simulink model "BuckeyeCurrent_Simulation"  (R2018a)
settings: Solver=FixedStepAuto  StartTime=0.0  StopTime=Inf  MinStep=0.01  RelTol=1e-3
undefined symbols (not defined in the file): A1, AIR, ambTemp_K, BATT_ELEC, BATT_OCV, BATT_THERMAL, C1, C2, Cell, COOLANT, cp, Elevation_Profile, EM, flowrate, hA1, k12, M, M2, MOT, RAD, soc0, V_pack_init, Velocity_Profile
libraries: simulink x3
(part 1 of 2)
settings Model: Creator=salyer.103  LastModifiedBy=Zach
settings SolverCC: ZeroCrossAlgorithm=Adaptive
settings CodeAppCC: StateflowObjectComments=on

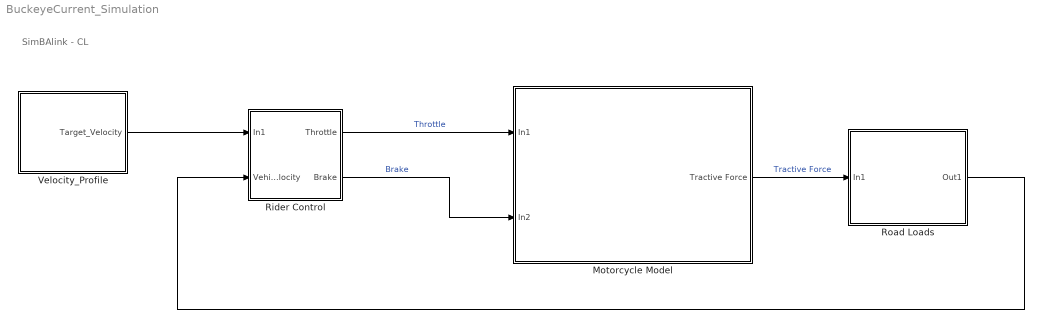
== system BuckeyeCurrent_Simulation ==
  note: SimBAlink - CL
  Motorcycle Model : Subsystem  mask{EM_MC_Selection=emrax268_pm150dz, SOC_max=0.95, SOC_min=0.10, Cell_Selection=Ideal, Wheel_Radius=0.3, Final_Drive_Eff=0.92, Max_Brake_Torque=4000, Total_Mass=330, b=0.728, h=0.72, g=9.81, p=1.4, mu_r=1, Front_Sprocket=21, Rear_Sprocket_FirstGear=40, Rear_Sprocket_SecondGear=40, Regen_Percent=0, Whl_Inertia=0, Transmission_Inertia=0}
      mask prompts: EM_MC_Selection "Motor & Controller Selection"; SOC_max "Maximum SOC"; SOC_min "Minimum SOC"; Cell_Selection "Cell Selection"; Wheel_Radius "Wheel Radius (m)"; Final_Drive_Eff "Efficiency of Drivetrain"; Max_Brake_Torque "Maximum Braking Torque (Nm)"; Total_Mass "Vehicle Total Mass (kg)"; b "Distance from Rear Wheel to CG (m)"; h "Height of CG from ground (m)"; g "Gravity (m/s2)"; p "Wheelbase (m)"; mu_r "Rear Wheel Coefficient of Friction"; Front_Sprocket "Front Sprocket Teeth"; Rear_Sprocket_FirstGear "Rear Sprocket 1st"; Rear_Sprocket_SecondGear "Rear Sprocket 2nd"; Regen_Percent "Percentage of Max Regen (%)"; Whl_Inertia "Wheel Inertia (kg-m2)"; Transmission_Inertia "Transmission Inertia (kg-m2)"
      mask init:
      | Initialize_Powertrain
      | Initialize_BatteryPack
      mask TypeOptions EM_MC_Selection: emrax268_pm150dz | RemyHVH25090s | emrax228_Twin | Ideal_TomegaCurve
      mask TypeOptions Cell_Selection: Ideal | Efest_IMR18650 | LG_INR18650HG2 | LG_INR18650MJ1 | SanPan_NCR18650GA
      mask Display:
      | directory = pwd;
      | image([pwd '\Mask Pictures\bike.jpg']);
  Rider Control : Subsystem  mask{kp=5, ki=0, kd=0}
      mask Display:
      | directory = pwd;
      | image([pwd '\Mask Pictures\helmet.jpg']);
  Road Loads : Subsystem  mask{rowA=1, Wind_Speed=0, Cda=0.38, ElevationProfile=IOM_ElevationProfile}
      mask prompts: rowA "Air Density"; Wind_Speed "Wind Speed (m/s)"; Cda "Cd * Frontal Area"; ElevationProfile "Course Elevation Profile"
      mask init:
      | Initialize_Elevation
      mask TypeOptions ElevationProfile: IOM_ElevationProfile | QuarterMile_ElevationProfile
  Velocity_Profile : Subsystem  mask{Circuit_Selection=IOM}
      mask prompts: Circuit_Selection "Circuit"
      mask init:
      | Initialize_Circuit
      mask TypeOptions Circuit_Selection: IOM | QuarterMile
      mask Display:
      | directory = pwd;
      | image([pwd '\Mask Pictures\VelocityProfile.png']);
  wires:
  Velocity_Profile/1(Target_Velocity) -> Rider Control/1(In1)
  Rider Control/1(Throttle) -> Motorcycle Model/1(In1)  "Throttle"
  Rider Control/2(Brake) -> Motorcycle Model/2(In2)  "Brake"
  Motorcycle Model/1(Tractive Force) -> Road Loads/1(In1)  "Tractive Force"
  Road Loads/1(Out1) -> Rider Control/2(Vehicle_Velocity)

== system BuckeyeCurrent_Simulation/Motorcycle Model ==
  note: When Rear Braking Strategy is added, will need to move pack energy req block
      | B/c negative torque applied gives regen to pack
      |
      | To determine actual applied torque prior to the wheel block we will  need to modulate torque based on
      | wheel slip from the rider model
  In1 : Inport
  In2 : Inport  Port=2
  Battery Pack : Subsystem
      mask Display:
      | directory = pwd;
      | image([directory '\Mask Pictures\pack.JPG']);
  Braking/Throttle Strategy : Subsystem
  Front Brakes : Subsystem
      mask Display:
      | directory = pwd;
      | image([directory '\Mask Pictures\motoBrake.JPG']);
  Front Wheel (Force Limits) : Subsystem
      mask Display:
      | directory = pwd;
      | image([directory '\Mask Pictures\frTire_pirelli.JPG']);
  Powertrain : Subsystem
      mask Display:
      | directory = pwd;
      | image([directory '\Mask Pictures\bike_powertrain.JPG']);
  Rear Brakes : Subsystem
      mask Display:
      | directory = pwd;
      | image([directory '\Mask Pictures\motoBrake.JPG']);
  Rear Wheel (Force Limits) : Subsystem
      mask Display:
      | directory = pwd;
      | image([directory '\Mask Pictures\rrTire_pirelli.JPG']);
  Sum : Sum  Inputs=+|+
  Sum1 : Sum  Inputs=++|
  To Workspace : ToWorkspace  VariableName=RearWhlForce  SampleTime=-1
  To Workspace1 : ToWorkspace  VariableName=FrontWhlForce  SaveFormat=Timeseries  SampleTime=-1
  Transmission : Subsystem
      mask Display:
      | directory = pwd;
      | image([directory '\Mask Pictures\gear.PNG']);
  Vehicle Parameters : Subsystem
  Tractive Force : Outport
  wires:
  Sum/1 -> Tractive Force/1  "Tractive Force"
  Powertrain/1(Motor Torque) -> Transmission/1(Motor Torque)
  Front Brakes/1(Front Wheel Torque) -> Front Wheel (Force Limits)/1(In1)
  Front Wheel (Force Limits)/1(Out2) -> Sum/1, To Workspace1/1
  Rear Wheel (Force Limits)/1(Out1) -> Sum/2, To Workspace/1
  In1/1 -> Braking/Throttle Strategy/1(In1)  "Throttle"
  Braking/Throttle Strategy/3(Out2) -> Powertrain/1(Throttle)
  In2/1 -> Braking/Throttle Strategy/2(In2)  "Brake"
  Braking/Throttle Strategy/1(Out3) -> Front Brakes/1(Throttle)
  Transmission/1(Out1) -> Sum1/2  "Wheel Torque"
  Rear Brakes/1(Front Wheel Torque) -> Sum1/1  "Rear Brake Torque"
  Sum1/1 -> Rear Wheel (Force Limits)/1(In1)  "Total Torque"
  Braking/Throttle Strategy/2(Out1) -> Rear Brakes/1(Throttle)
  Powertrain/2(Out1) -> Battery Pack/1(In1)  "Power Request"
  Battery Pack/1(Power Limit) -> Powertrain/2(df\)  "Power Limit"
  Battery Pack/2(Power Limit1) -> Powertrain/3(df\1)  "Terminal Voltage"

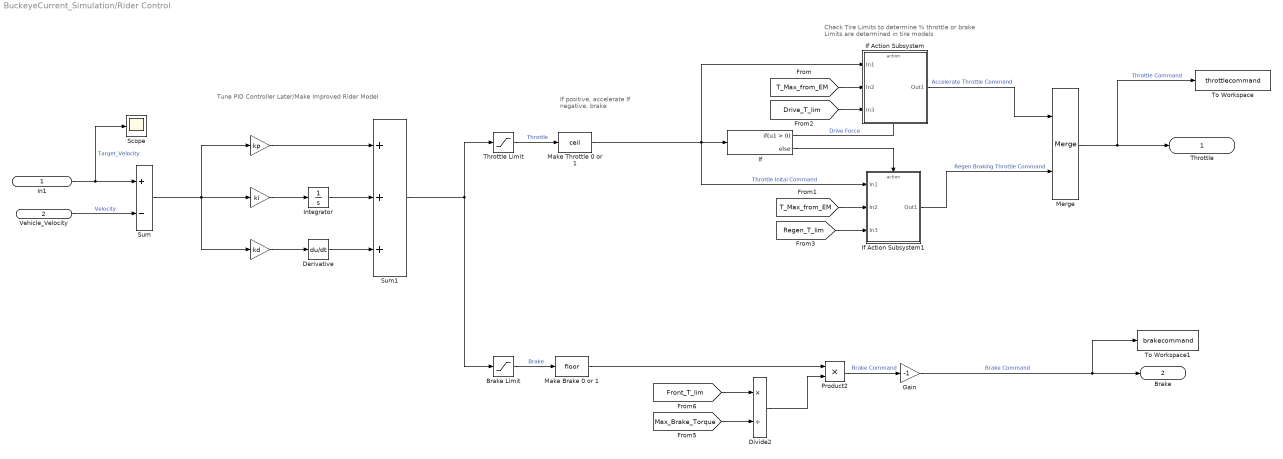
== system BuckeyeCurrent_Simulation/Rider Control ==
  note: Check Tire Limits to determine % throttle or brake
      | Limits are determined in tire models
  note: If positive, accelerate
      | If negative, brake
  note: Tune PID Controller Later/Make Improved Rider Model
  In1 : Inport
  Vehicle_Velocity : Inport  Port=2
  " " : Gain  Gain=ki
  "  " : Gain  Gain=kp
  "   " : Gain  Gain=kd
  Brake Limit : Saturate  UpperLimit=0  LowerLimit=-1  ZeroCross=off
  Derivative : Derivative
  Divide2 : Product  Inputs=*/
  Gain : Gain  Gain=-1
  If : If
  If Action Subsystem : Subsystem  TreatAsAtomicUnit=on
  If Action Subsystem1 : Subsystem  TreatAsAtomicUnit=on
  Integrator : Integrator
  Make Brake 0 or 1 : Rounding
  Make Throttle 0 or 1 : Rounding  Operator=ceil
  Merge : Merge
  Product2 : Product
  Scope : Scope
  Sum : Sum  Inputs=+-
  Sum1 : Sum  Inputs=+++
  Throttle Limit : Saturate  UpperLimit=1  LowerLimit=0  ZeroCross=off
  To Workspace : ToWorkspace  VariableName=throttlecommand  SampleTime=-1
  To Workspace1 : ToWorkspace  VariableName=brakecommand  SampleTime=-1
  Throttle : Outport
  Brake : Outport  Port=2
  wires:
  Vehicle_Velocity/1 -> Sum/2  "Velocity"
  In1/1 -> Scope/1, Sum/1  "Target_Velocity"
  "  "/1 -> Sum1/1
  Sum/1 -> "  "/1, " "/1, "   "/1
  Throttle Limit/1 -> Make Throttle 0 or 1/1  "Throttle"
  " "/1 -> Integrator/1
  Integrator/1 -> Sum1/2
  "   "/1 -> Derivative/1
  Derivative/1 -> Sum1/3
  Sum1/1 -> Brake Limit/1, Throttle Limit/1
  Brake Limit/1 -> Make Brake 0 or 1/1  "Brake"
  Make Throttle 0 or 1/1 -> If Action Subsystem/1(In1), If Action Subsystem1/1(In1), If/1  "Throttle Inital Command"
  Merge/1 -> To Workspace/1, Throttle/1  "Throttle Command"
  [Max_Brake_Torque] -> Divide2/2
  [Front_T_lim] -> Divide2/1
  Divide2/1 -> Product2/2
  Make Brake 0 or 1/1 -> Product2/1
  Gain/1 -> To Workspace1/1, Brake/1  "Brake Command"
  If Action Subsystem/1(Out1) -> Merge/1  "Accelerate Throttle Command"
  If Action Subsystem1/1(Out1) -> Merge/2  "Regen Braking Throttle Command"
  [T_Max_from_EM] -> If Action Subsystem/2(In2)
  [T_Max_from_EM] -> If Action Subsystem1/2(In2)
  [Drive_T_lim] -> If Action Subsystem/3(In3)
  [Regen_T_lim] -> If Action Subsystem1/3(In3)
  If/1 -> If Action Subsystem/Action  "Drive Force"
  If/2 -> If Action Subsystem1/Action
  Product2/1 -> Gain/1  "Brake Command"

== system BuckeyeCurrent_Simulation/Road Loads ==
  In1 : Inport
  Enviornment : Subsystem
  To Workspace : ToWorkspace  VariableName=Vehicle_Velocity  SampleTime=-1
      settings: Save2DSignal=2-D array (concatenate along first dimension)
  To Workspace1 : ToWorkspace  VariableName=resistanceforce  SampleTime=-1
      settings: Save2DSignal=2-D array (concatenate along first dimension)
  Vehicle Loads : Subsystem
  Vehicle_speed_Calculation : Subsystem
  Out1 : Outport
  tag scope: Vehicle_Velocity_ms=global
  wires:
  In1/1 -> Vehicle_speed_Calculation/1(In1)  "Tractive Force"
  Vehicle_speed_Calculation/1(F (N)1) -> To Workspace/1, Out1/1, [Vehicle_Velocity_ms]  "Velocity"
  Vehicle Loads/1(F (N)) -> To Workspace1/1, Vehicle_speed_Calculation/2(In3)

== system BuckeyeCurrent_Simulation/Velocity_Profile ==
  Constant : Constant  Value=Velocity_Profile.distance(end)
  Relational Operator1 : RelationalOperator  RndMeth=Nearest  InputSameDT=on
  Stop Simulation : Stop
  To Workspace : ToWorkspace  VariableName=Target_Velocity  SampleTime=-1
  Vehicle_Target_Speed : Lookup  InputValues=Velocity_Profile.distance  Table=Velocity_Profile.velocity  LookUpMeth=Interpolation-Use End Values  SaturateOnIntegerOverflow=on
  Target_Velocity : Outport
  wires:
  Vehicle_Target_Speed/1 -> To Workspace/1, Target_Velocity/1  "Target_Velocity"
  Constant/1 -> Relational Operator1/2
  Relational Operator1/1 -> Stop Simulation/1
  [Distance_Total_m] -> Relational Operator1/1, Vehicle_Target_Speed/1

== system BuckeyeCurrent_Simulation/Motorcycle Model/Battery Pack ==
  In1 : Inport
  0th Order Cell Model : Subsystem
  Constant : Constant  Value=Cell.Np
  Constant2 : Constant  Value=Cell.Ns
  Constant3 : Constant  Value=Cell.Nt
  "Current Lim, 1st Order ECM, Thermal, Regen" : Subsystem  Commented=on
  Integrator : Integrator
  Multiply : Product  Inputs=*/
  Multiply1 : Product  Inputs=*/
  Multiply{2..4,6} (4 alike) : Product
  To Workspace1 : ToWorkspace  VariableName=P_pack  SampleTime=-1
      settings: Save2DSignal=2-D array (concatenate along first dimension)
  To Workspace2 : ToWorkspace  VariableName=E_pack  SampleTime=-1
      settings: Save2DSignal=2-D array (concatenate along first dimension)
  To Workspace3 : ToWorkspace  VariableName=I_pack  SampleTime=-1
      settings: Save2DSignal=2-D array (concatenate along first dimension)
  To Workspace4 : ToWorkspace  VariableName=SOC  SampleTime=-1
      settings: Save2DSignal=2-D array (concatenate along first dimension)
  To Workspace5 : ToWorkspace  VariableName=V_pack  SampleTime=-1
      settings: Save2DSignal=2-D array (concatenate along first dimension)
  To Workspace6 : ToWorkspace  VariableName=Q_pack  SampleTime=-1
      settings: Save2DSignal=2-D array (concatenate along first dimension)
  W to kW : Gain  Gain=1/1000
  kW-s to kW-h : Gain  Gain=1/3600
  Power Limit : Outport
  Power Limit1 : Outport  Port=2
  wires:
  kW-s to kW-h/1 -> To Workspace2/1
  Integrator/1 -> kW-s to kW-h/1  "Energy"
  W to kW/1 -> Integrator/1, To Workspace1/1
  Multiply1/1 -> 0th Order Cell Model/1(Current [A])
  Multiply/1 -> Multiply1/1, Multiply6/1, To Workspace3/1
  Constant/1 -> Multiply1/2
  In1/1 -> Multiply/1  "Inverter_Power_Request"
  0th Order Cell Model/1(SOC [-]) -> To Workspace4/1
  0th Order Cell Model/3(Heat Generation [W]) -> Multiply2/1
  Constant3/1 -> Multiply2/2, Multiply4/2
  0th Order Cell Model/4(" Cell Voltage [V]") -> Multiply3/1
  Constant2/1 -> Multiply3/2
  Multiply3/1 -> Power Limit1/1, To Workspace5/1, Multiply6/2, Multiply/2  "Terminal Voltage"
  Multiply2/1 -> To Workspace6/1
  Multiply4/1 -> Power Limit/1  "Power Limit"
  0th Order Cell Model/2(Power Limit [W]) -> Multiply4/1
  Multiply6/1 -> W to kW/1

== system BuckeyeCurrent_Simulation/Motorcycle Model/Braking//Throttle Strategy ==
  note: Notes:
      | -No Rear Brake currently being used, no point in using it until we have a better rider model
      | -If throttle = 0, then switch to -1 to request negative torque
      | -Need to add a limit to rear brake force based on friction
  In1 : Inport
  In2 : Inport  Port=2
  Constant : Constant  Value=0
  Constant1 : Constant  Value=-1
  Gain : Gain
  Switch : Switch  Criteria=u2 > Threshold
  Out3 : Outport
  Out1 : Outport  Port=2
  Out2 : Outport  Port=3
  wires:
  Constant/1 -> Out1/1  "Rear Brake Request"
  In1/1 -> Switch/1, Switch/2  "Throttle Request"
  In2/1 -> Gain/1  "Brake Request"
  Gain/1 -> Out3/1  "Front Brake Request"
  Constant1/1 -> Switch/3
  Switch/1 -> Out2/1  "Torque Request"

== system BuckeyeCurrent_Simulation/Motorcycle Model/Front Brakes ==
  Throttle : Inport
  Multiply : Product  Inputs=**
  Front Wheel Torque : Outport
  wires:
  Throttle/1 -> Multiply/1  "Brake"
  [Max_Brake_Torque] -> Multiply/2
  Multiply/1 -> Front Wheel Torque/1  "Front Wheel Torque"

== system BuckeyeCurrent_Simulation/Motorcycle Model/Front Wheel (Force Limits) ==
  In1 : Inport
  Divide : Product  Inputs=*/
  Divide1 : Product  Inputs=**
  Dynamic Front Wheel Load * mu : Fcn  Expr=-mu_r*Total_Mass*g*b/p + u(1)*h/p
  Memory : Memory
  Memory1 : Memory
  Min : MinMax  Inputs=2
  Stoppie Limit Brake Force : Constant  Value=-Total_Mass*g*(p-b)/h
  Sum : Sum  Inputs=|++
  Sum1 : Sum
  Out2 : Outport
  tag scope: Front_Brake_Force=global, Front_T_lim=global
  wires:
  In1/1 -> Divide/1  "Front Wheel Torque"
  Divide/1 -> Out2/1, [Front_Brake_Force]  "Tractive Force"
  [Fr_Wheel_Radius] -> Divide/2
  Sum1/1 -> Dynamic Front Wheel Load * mu/1
  Dynamic Front Wheel Load * mu/1 -> Min/1
  Stoppie Limit Brake Force/1 -> Min/2
  [Front_Brake_Force] -> Memory/1
  Memory/1 -> Sum1/1
  Memory1/1 -> Sum1/2
  Min/1 -> Divide1/1
  Divide1/1 -> [Front_T_lim]
  [Fr_Wheel_Radius] -> Divide1/2
  Sum/1 -> Memory1/1
  [Regen_Brake_Force] -> Sum/1
  [Rear_Brake_Force] -> Sum/2

== system BuckeyeCurrent_Simulation/Motorcycle Model/Powertrain ==
  note: Note: Once thermal models are calibrated, the torque request will pass through those models to see if thermal is limiting power
      | -For now, assuming ideal motor and inverter
  Throttle : Inport
  df\ : Inport  Port=2
  df\1 : Inport  Port=3
  Divide : Product  Inputs=*/
  Gain : Gain  Gain=2*pi/60
  Integrator : Integrator
  Powertrain Mechanical : Subsystem
  Powertrain Thermal Model : Subsystem  Commented=on
  Product : Product
  Sum : Sum  Inputs=|-+
  To Workspace : ToWorkspace  VariableName=Heat_Energy_J  SampleTime=-1
  Motor Torque : Outport
  Out1 : Outport  Port=2
  wires:
  Throttle/1 -> Powertrain Mechanical/1(In1)  "Throttle"
  Powertrain Thermal Model/1(Out1) -> ?  "Motor Torque (With Possible Thermal Limtis)"
  Powertrain Thermal Model/2(Out2) -> ?  "Inverter_P_Request"
  Powertrain Mechanical/1(Out1) -> Product/1, Motor Torque/1  "Motor Torque"
  Powertrain Mechanical/2(EM RPM) -> Gain/1
  Gain/1 -> Product/2  "rad/s"
  Product/1 -> Sum/1, Divide/1  "Motor_Power_req"
  [EM_eff] -> Divide/2
  Divide/1 -> Sum/2, Out1/1  "Total_Power"
  Sum/1 -> Integrator/1  "heat_power_W"
  Integrator/1 -> To Workspace/1
  df\/1 -> Powertrain Mechanical/2(Power Limit)  "Power Limit"
  df\1/1 -> Powertrain Mechanical/3(Terminal Voltage)  "Terminal Voltage"

== system BuckeyeCurrent_Simulation/Motorcycle Model/Rear Brakes ==
  Throttle : Inport
  Multiply : Product  Inputs=**
  Front Wheel Torque : Outport
  tag scope: Rear_Brake_Force=global
  wires:
  Throttle/1 -> Multiply/1  "Brake"
  [Max_Brake_Torque] -> Multiply/2
  Multiply/1 -> [Rear_Brake_Force], Front Wheel Torque/1  "Rear Wheel Torque"

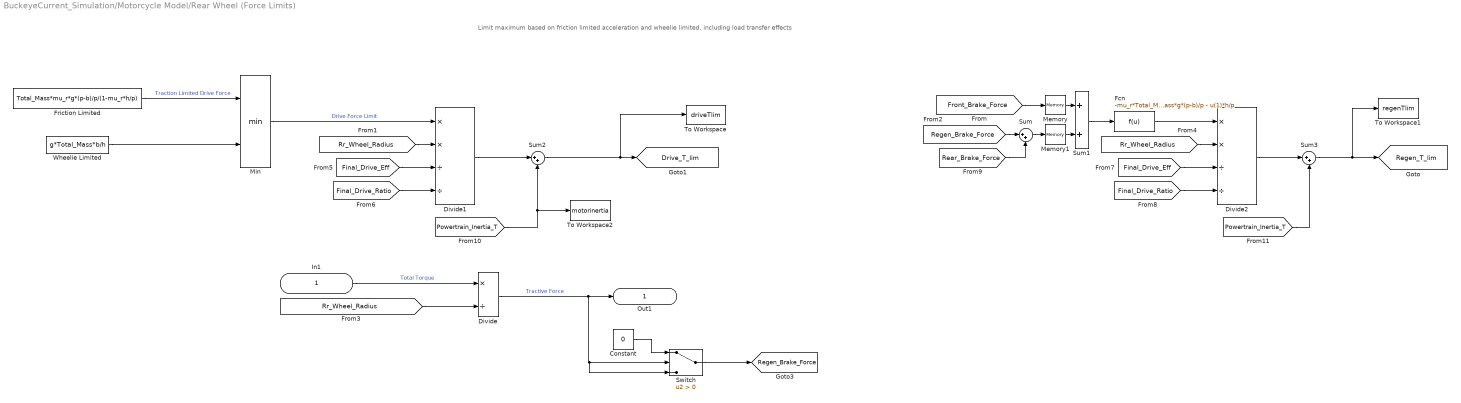
== system BuckeyeCurrent_Simulation/Motorcycle Model/Rear Wheel (Force Limits) ==
  note: Limit maximum based on friction limited acceleration and wheelie limited, including load transfer effects
  In1 : Inport
  Constant : Constant  Value=0
  Divide : Product  Inputs=*/
  Divide1 : Product  Inputs=**//
  Divide2 : Product  Inputs=**//
  Fcn : Fcn  Expr=-mu_r*Total_Mass*g*(p-b)/p - u(1)*h/p
  Friction Limited : Constant  Value=Total_Mass*mu_r*g*(p-b)/p/(1-mu_r*h/p)
  Memory : Memory
  Memory1 : Memory
  Min : MinMax  Inputs=2
  Sum : Sum  Inputs=|++
  Sum1 : Sum
  Sum2 : Sum  Inputs=|++
  Sum3 : Sum  Inputs=|++
  Switch : Switch  Criteria=u2 > Threshold
  To Workspace : ToWorkspace  VariableName=driveTlim  SampleTime=-1
  To Workspace1 : ToWorkspace  VariableName=regenTlim  SampleTime=-1
  To Workspace2 : ToWorkspace  VariableName=motorinertia  SampleTime=-1
  Wheelie Limited : Constant  Value=g*Total_Mass*b/h
  Out1 : Outport
  tag scope: Drive_T_lim=global, Regen_Brake_Force=global, Regen_T_lim=global
  wires:
  [Rr_Wheel_Radius] -> Divide/2
  Wheelie Limited/1 -> Min/2
  In1/1 -> Divide/1  "Total Torque"
  Divide/1 -> Switch/3, Switch/2, Out1/1  "Tractive Force"
  Sum1/1 -> Fcn/1
  Friction Limited/1 -> Min/1  "Traction Limited Drive Force"
  Min/1 -> Divide1/1  "Drive Force Limit"
  [Front_Brake_Force] -> Memory/1
  Memory/1 -> Sum1/1
  Memory1/1 -> Sum1/2
  Switch/1 -> [Regen_Brake_Force]
  Sum2/1 -> To Workspace/1, [Drive_T_lim]
  Fcn/1 -> Divide2/1
  Constant/1 -> Switch/1
  [Rr_Wheel_Radius] -> Divide1/2
  [Final_Drive_Eff] -> Divide1/3
  [Final_Drive_Ratio] -> Divide1/4
  [Final_Drive_Ratio] -> Divide2/4
  [Rr_Wheel_Radius] -> Divide2/2
  [Final_Drive_Eff] -> Divide2/3
  Sum/1 -> Memory1/1
  [Regen_Brake_Force] -> Sum/1
  [Rear_Brake_Force] -> Sum/2
  Divide1/1 -> Sum2/1
  [Powertrain_Inertia_T] -> To Workspace2/1, Sum2/2
  Divide2/1 -> Sum3/1
  Sum3/1 -> To Workspace1/1, [Regen_T_lim]
  [Powertrain_Inertia_T] -> Sum3/2

== system BuckeyeCurrent_Simulation/Motorcycle Model/Transmission ==
  note: Actual Motor RPM Depends on what gear we're in
  Motor Torque : Inport
  "CONVERT TO whl RPM " : Gain  Gain=60
  Calc wheel circumference : Gain  Gain=2*3.14
  Derivative : Derivative
  Gain : Gain  Gain=2*pi/60
  "Gearbox " : Subsystem
  To Workspace : ToWorkspace  VariableName=FinalDriveRatio  SampleTime=-1
      settings: Save2DSignal=2-D array (concatenate along first dimension)
  To Workspace1 : ToWorkspace  VariableName=RearWheelTorque  SampleTime=-1
      settings: Save2DSignal=2-D array (concatenate along first dimension)
  "convert to whl rev per sec " : Product  Inputs=*/
  "product rpm " : Product  Inputs=**
  product rpm 1 : Product  Inputs=**
  product rpm 2 : Product  Inputs=**
  Out1 : Outport
  tag scope: EM_RPM=global, EM_RPM_1st=global, EM_RPM_2nd=global, EM_acc=global
  wires:
  "Gearbox "/2(Out1) -> To Workspace1/1, Out1/1  "Rear Wheel Torque"
  Calc wheel circumference/1 -> "convert to whl rev per sec "/2
  [Vehicle_Velocity_ms] -> "convert to whl rev per sec "/1
  [Rr_Wheel_Radius] -> Calc wheel circumference/1
  "convert to whl rev per sec "/1 -> "CONVERT TO whl RPM "/1
  "product rpm "/1 -> Gain/1, [EM_RPM]
  Motor Torque/1 -> "Gearbox "/1(In1)  "Motor Torque"
  "CONVERT TO whl RPM "/1 -> product rpm 2/2, product rpm 1/2, "product rpm "/1
  [Final_Drive_Ratio_1st] -> product rpm 1/1
  [Final_Drive_Ratio_2nd] -> product rpm 2/1
  product rpm 1/1 -> [EM_RPM_1st]
  product rpm 2/1 -> [EM_RPM_2nd]
  "Gearbox "/1(Out2) -> To Workspace/1, "product rpm "/2
  Gain/1 -> Derivative/1  "EMl speed (rad/s)"
  Derivative/1 -> [EM_acc]

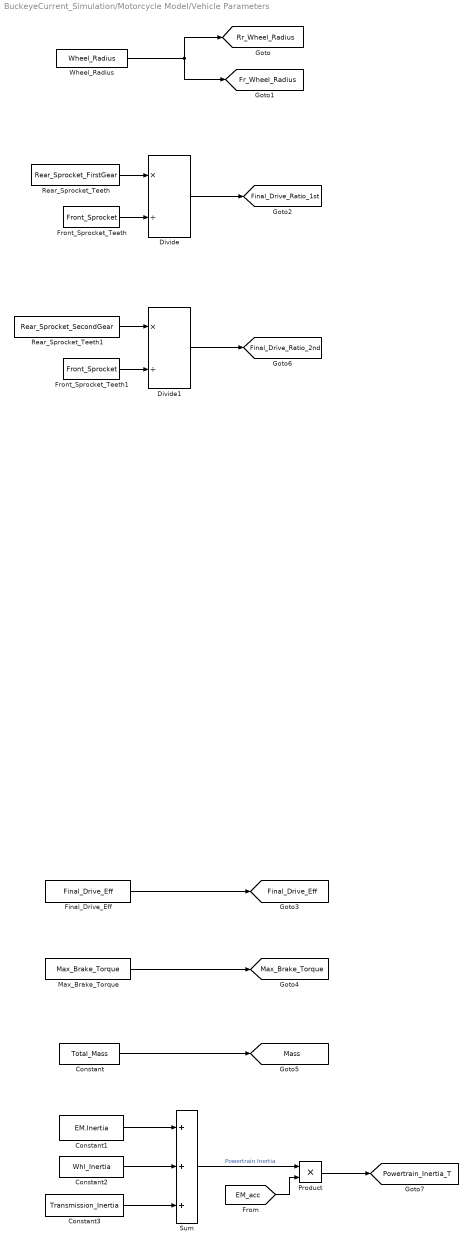
== system BuckeyeCurrent_Simulation/Motorcycle Model/Vehicle Parameters ==
  Constant : Constant  Value=Total_Mass
  Constant1 : Constant  Value=EM.Inertia
  Constant2 : Constant  Value=Whl_Inertia
  Constant3 : Constant  Value=Transmission_Inertia
  Divide : Product  Inputs=*/
  Divide1 : Product  Inputs=*/
  Final_Drive_Eff : Constant  Value=Final_Drive_Eff
  Front_Sprocket_Teeth : Constant  Value=Front_Sprocket
  Front_Sprocket_Teeth1 : Constant  Value=Front_Sprocket
  Max_Brake_Torque : Constant  Value=Max_Brake_Torque
  Product : Product
  Rear_Sprocket_Teeth : Constant  Value=Rear_Sprocket_FirstGear
  Rear_Sprocket_Teeth1 : Constant  Value=Rear_Sprocket_SecondGear
  Sum : Sum  Inputs=+++
  Wheel_Radius : Constant  Value=Wheel_Radius
  tag scope: Final_Drive_Eff=global, Final_Drive_Ratio_1st=global, Final_Drive_Ratio_2nd=global, Fr_Wheel_Radius=global, Mass=global, Max_Brake_Torque=global, Powertrain_Inertia_T=global, Rr_Wheel_Radius=global
  wires:
  Wheel_Radius/1 -> [Rr_Wheel_Radius], [Fr_Wheel_Radius]
  Front_Sprocket_Teeth/1 -> Divide/2
  Rear_Sprocket_Teeth/1 -> Divide/1
  Final_Drive_Eff/1 -> [Final_Drive_Eff]
  Max_Brake_Torque/1 -> [Max_Brake_Torque]
  Constant/1 -> [Mass]
  Divide/1 -> [Final_Drive_Ratio_1st]
  Divide1/1 -> [Final_Drive_Ratio_2nd]
  Rear_Sprocket_Teeth1/1 -> Divide1/1
  Front_Sprocket_Teeth1/1 -> Divide1/2
  Constant1/1 -> Sum/1
  Constant2/1 -> Sum/2
  Constant3/1 -> Sum/3
  Sum/1 -> Product/1  "Powertrain Inertia"
  [EM_acc] -> Product/2
  Product/1 -> [Powertrain_Inertia_T]

== system BuckeyeCurrent_Simulation/Rider Control/If Action Subsystem ==
  In1 : Inport
  In2 : Inport  Port=2
  In3 : Inport  Port=3
  Action Port : ActionPort  ActionType=then
  Divide : Product  Inputs=*/
  Product : Product
  Throttle Limit1 : Saturate  UpperLimit=1  LowerLimit=0  ZeroCross=off
  Out1 : Outport
  wires:
  Throttle Limit1/1 -> Out1/1
  Divide/1 -> Product/1
  In3/1 -> Divide/1
  In2/1 -> Divide/2  "T_Max_EM"
  In1/1 -> Product/2  "Drive Force"
  Product/1 -> Throttle Limit1/1

== system BuckeyeCurrent_Simulation/Rider Control/If Action Subsystem1 ==
  In1 : Inport
  In2 : Inport  Port=2
  In3 : Inport  Port=3
  Action Port : ActionPort  ActionType=else
  Constant : Constant  Value=-1
  Divide1 : Product  Inputs=*/
  Product1 : Product
  Sum2 : Sum  Inputs=|++
  Throttle Limit2 : Saturate  UpperLimit=0  LowerLimit=-1  ZeroCross=off
  Out1 : Outport
  wires:
  Throttle Limit2/1 -> Out1/1
  In1/1 -> Sum2/1
  Sum2/1 -> Product1/1  "Set throttle to -1"
  Constant/1 -> Sum2/2
  In3/1 -> Divide1/1
  Product1/1 -> Throttle Limit2/1
  In2/1 -> Divide1/2  "T_Max_EM"
  Divide1/1 -> Product1/2

== system BuckeyeCurrent_Simulation/Road Loads/Enviornment ==
  Constant : Constant  Value=Cda
  Constant1 : Constant  Value=Wind_Speed
  Constant4 : Constant  Value=rowA
  tag scope: Cda=global, Row_Air=global, Wind_Speed=global
  wires:
  Constant1/1 -> [Wind_Speed]  "wind speed"
  Constant4/1 -> [Row_Air]  "air density"
  Constant/1 -> [Cda]

== system BuckeyeCurrent_Simulation/Road Loads/Vehicle Loads ==
  Aerodynamic  Drag : Subsystem
  Grade Force : Subsystem
  Roll Force : Subsystem
  Sum4 : Sum  Inputs=+++
  To Workspace : ToWorkspace  VariableName=gradeforce  SampleTime=-1
  F (N) : Outport
  wires:
  Sum4/1 -> F (N)/1  "Road Load (N)"
  Roll Force/1(Power_roll) -> Sum4/3
  Aerodynamic  Drag/1(Drag Power) -> Sum4/2
  Grade Force/1(Drag Power) -> To Workspace/1, Sum4/1  "Grade Force"

== system BuckeyeCurrent_Simulation/Road Loads/Vehicle_speed_Calculation ==
  In1 : Inport
  In3 : Inport  Port=2
  Divide : Product  Inputs=*/
  Integrator Limited : Integrator  LimitOutput=on  LowerSaturationLimit=0
  Integrator Limited1 : Integrator  LimitOutput=on  LowerSaturationLimit=0
  Sum : Sum  Inputs=+-
  To Workspace : ToWorkspace  VariableName=Vehicle_Distance  SampleTime=-1
      settings: Save2DSignal=2-D array (concatenate along first dimension)
  F (N)1 : Outport
  tag scope: Distance_Total_m=global
  wires:
  Sum/1 -> Divide/1  "Net_Force"
  Divide/1 -> Integrator Limited/1  "Vehicle_Acceleration"
  In1/1 -> Sum/1
  [Mass] -> Divide/2
  In3/1 -> Sum/2
  Integrator Limited/1 -> F (N)1/1, Integrator Limited1/1  "vehicle_speed"
  Integrator Limited1/1 -> To Workspace/1, [Distance_Total_m]  "distance"

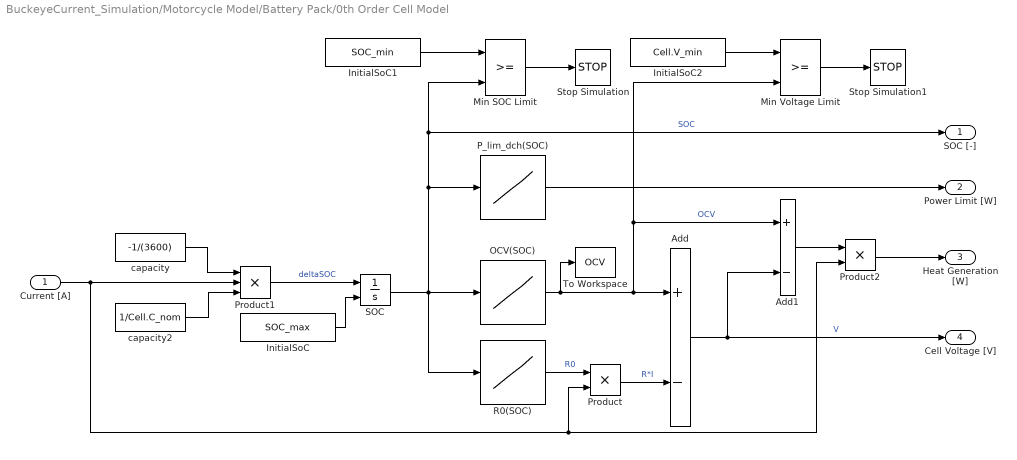
== system BuckeyeCurrent_Simulation/Motorcycle Model/Battery Pack/0th Order Cell Model ==
  Current [A] : Inport
  Add : Sum  Inputs=+-
  Add1 : Sum  Inputs=+-
  InitialSoC : Constant  Value=SOC_max
  InitialSoC1 : Constant  Value=SOC_min
  InitialSoC2 : Constant  Value=Cell.V_min
  Min SOC Limit : RelationalOperator  OutDataTypeStr=boolean  RndMeth=Simplest
  Min Voltage Limit : RelationalOperator  OutDataTypeStr=boolean  RndMeth=Simplest
  OCV(SOC) : Lookup_n-D  NumberOfTableDimensions=1  BreakpointsForDimension1=Cell.SOC_dch  Table=Cell.OCV_dch  RndMeth=Simplest  InputSameDT=on
  P_lim_dch(SOC) : Lookup_n-D  NumberOfTableDimensions=1  BreakpointsForDimension1=Cell.SOC_dch  Table=Cell.P_lim_dch  RndMeth=Simplest  InputSameDT=on
  Product : Product  RndMeth=Zero
  Product1 : Product  Inputs=3  RndMeth=Zero
  Product2 : Product  RndMeth=Zero
  R0(SOC) : Lookup_n-D  NumberOfTableDimensions=1  BreakpointsForDimension1=Cell.SOC_dch  Table=Cell.R_dch  RndMeth=Simplest  InputSameDT=on
  SOC : Integrator  InitialConditionSource=external  InitialCondition=1
  Stop Simulation : Stop
  Stop Simulation1 : Stop
  To Workspace : ToWorkspace  VariableName=OCV  SampleTime=-1
  capacity : Constant  Value=-1/(3600)
  capacity2 : Constant  Value=1/Cell.C_nom
  SOC [-] : Outport
  Power Limit [W] : Outport  Port=2
  Heat Generation [W] : Outport  Port=3
  " Cell Voltage [V]" : Outport  Port=4
  wires:
  InitialSoC/1 -> SOC/2
  Current [A]/1 -> Product/2, Product2/2, Product1/2
  capacity2/1 -> Product1/3
  OCV(SOC)/1 -> To Workspace/1, Min Voltage Limit/2, Add1/1, Add/1  "OCV"
  Product/1 -> Add/2  "R*I"
  Add/1 -> Add1/2, " Cell Voltage [V]"/1  "V"
  capacity/1 -> Product1/1
  Product1/1 -> SOC/1  "deltaSOC"
  SOC/1 -> Min SOC Limit/2, SOC [-]/1, P_lim_dch(SOC)/1, R0(SOC)/1, OCV(SOC)/1  "SOC"
  Add1/1 -> Product2/1
  Product2/1 -> Heat Generation [W]/1
  R0(SOC)/1 -> Product/1  "R0"
  P_lim_dch(SOC)/1 -> Power Limit [W]/1
  InitialSoC1/1 -> Min SOC Limit/1
  Min SOC Limit/1 -> Stop Simulation/1
  Min Voltage Limit/1 -> Stop Simulation1/1
  InitialSoC2/1 -> Min Voltage Limit/1

== system BuckeyeCurrent_Simulation/Motorcycle Model/Battery Pack/Current Lim, 1st Order ECM, Thermal, Regen ==
  In1 : Inport
  Battery Parameters Calculation : Subsystem
      mask Display:
      | color('blue');
      | fprintf('Battery Parameters Calculation')
  Battery to Cell : Subsystem
      mask Display:
      | color('blue');
      | fprintf('Battery to Cell')
  Cell : Subsystem
      mask Display:
      | color('blue');
      | fprintf('Cell: 1st Order Electrical Model')
  Cell to Batt : Subsystem
      mask Display:
      | color('blue');
      | fprintf('Cell to Battery')
  "Current Limiter " : simulink/Discontinuities/Saturation Dynamic  OutMin=[]  OutMax=[]  OutDataTypeStr=Inherit: Same as second input  OutDataType=sfix(16)  OutScaling=2^-10  DoSatur=off
  Divide : Product  Inputs=/*
  Gain1 : Gain  Gain=-1
  Memory : Memory
  Sum : Sum
  Thermal Dynamics : Subsystem
      mask Display:
      | color('blue');
      | fprintf('Battery Thermal')
  tag scope: P_from_Battery=global
  wires:
  Memory/1 -> "Current Limiter "/2
  Cell to Batt/1(Out1) -> Divide/1
  Cell/1(Out1) -> Cell to Batt/1(In1)
  Divide/1 -> Memory/1  "I_Batt_Req"
  In1/1 -> Sum/2  "Inverter_Power_Request"
  Cell/2(Out2) -> Cell to Batt/2(In2)
  "Current Limiter "/1 -> Battery Parameters Calculation/1(current1), Battery to Cell/1(In1)  "I_Batt"
  Battery to Cell/1(Out1) -> Cell/1(In2)
  [DClink_Fuse] -> Gain1/1
  [DClink_Fuse] -> "Current Limiter "/1
  Gain1/1 -> "Current Limiter "/3
  Cell to Batt/2(Out3) -> [P_from_Battery]
  Sum/1 -> Divide/2  "P_Req"
  ? -> Sum/1  "P_Heat_Pack"

== system BuckeyeCurrent_Simulation/Motorcycle Model/Powertrain/Powertrain Mechanical ==
  note: Apply max torque (sign will depend on if throttle is positive or negative - regen or accelerate)
      | Apply gain for regen percentage to decrease from max torque is desired
  In1 : Inport
  Power Limit : Inport  Port=2
  Terminal Voltage : Inport  Port=3
  Constant : Constant  Value=EM.kv
  Divide : Product  Inputs=**
  Divide1 : Product  Inputs=*/
  EM Max Torque Curve : Lookup  InputValues=EM.N_RPM  Table=EM.T_max_Peak  LookUpMeth=Interpolation-Use End Values  SaturateOnIntegerOverflow=on
  EM-EffMap : Lookup_n-D  BreakpointsForDimension1=EM.TorqueLookup  BreakpointsForDimension2=EM.N_RPM  Table=EM.eff_map  InternalRulePriority=Speed  RndMeth=Simplest  InputSameDT=on
  Gain : Gain  Gain=Regen_Percent/100
  Gain1 : Gain  Gain=2*pi/60
  Memory : Memory  InitialCondition=V_pack_init
  Multiply : Product
  RPM Limit : simulink/Discontinuities/Saturation Dynamic  OutMin=[]  OutMax=[]  OutDataTypeStr=Inherit: Same as second input  OutDataType=fixdt(1, 16)  OutScaling=2^-10  DoSatur=off
  Switch : Switch  Criteria=u2 > Threshold
  To Workspace : ToWorkspace  VariableName=EM_RPM  SampleTime=-1
      settings: Save2DSignal=2-D array (concatenate along first dimension)
  To Workspace2 : ToWorkspace  VariableName=motorT  SampleTime=-1
  Torque Limit : simulink/Discontinuities/Saturation Dynamic  OutMin=[]  OutMax=[]  OutDataTypeStr=Inherit: Same as second input  OutDataType=fixdt(1, 16)  OutScaling=2^-10  DoSatur=off
  Out1 : Outport
  EM RPM : Outport  Port=2
  tag scope: EM_eff=global, T_Max_from_EM=global
  wires:
  Gain/1 -> Switch/3
  Switch/1 -> Out1/1  "Torque"
  Divide/1 -> Switch/1, Switch/2, Gain/1, To Workspace2/1, EM-EffMap/1  "Motor Torque"
  In1/1 -> Divide/1  "Throttle"
  [T_Max_from_EM] -> Divide/2
  EM-EffMap/1 -> [EM_eff]  "EM_eff"
  [EM_RPM] -> EM-EffMap/2
  Power Limit/1 -> Divide1/1  "Power Limit"
  Constant/1 -> Multiply/1
  Multiply/1 -> RPM Limit/1
  [EM_RPM] -> RPM Limit/2, RPM Limit/3  "EM_RPM"
  RPM Limit/1 -> EM Max Torque Curve/1, Gain1/1, EM RPM/1, To Workspace/1  "EM RPM"
  EM Max Torque Curve/1 -> Torque Limit/2, Torque Limit/3  "Max Torque"
  Gain1/1 -> Divide1/2  "rad/s"
  Divide1/1 -> Torque Limit/1
  Torque Limit/1 -> [T_Max_from_EM]
  Memory/1 -> Multiply/2
  Terminal Voltage/1 -> Memory/1  "Terminal Voltage"

== system BuckeyeCurrent_Simulation/Motorcycle Model/Powertrain/Powertrain Thermal Model ==
  In1 : Inport
  In2 : Inport  Port=2
  Constant : Constant
  EMRAX Motor Thermal Model : Subsystem
  "Limit Torque/Power if neccessary for thermal " : Subsystem
  Radiator Thermal Model : Subsystem
  Rinehart Inverter Thermal Model : Subsystem
  To Workspace1 : ToWorkspace  VariableName=Stator_Temp  SaveFormat=Timeseries  SampleTime=-1
  To Workspace3 : ToWorkspace  VariableName=Rotor_Temp  SaveFormat=Timeseries  SampleTime=-1
  To Workspace4 : ToWorkspace  VariableName=Motor_Mounting_Temp  SaveFormat=Timeseries  SampleTime=-1
  Out1 : Outport
  Out2 : Outport  Port=2
  wires:
  In2/1 -> EMRAX Motor Thermal Model/1(Motor Speed [rpm])  "RPM"
  In1/1 -> EMRAX Motor Thermal Model/2(Motor Torque [Nm])  "Torque"
  Constant/1 -> EMRAX Motor Thermal Model/3(Motor ON Flag [-])
  EMRAX Motor Thermal Model/2(T_mass_2 [K]) -> To Workspace3/1
  EMRAX Motor Thermal Model/1(T_mass_1 [K]) -> To Workspace1/1
  EMRAX Motor Thermal Model/4(T_mass_3 [K]1) -> To Workspace4/1
  [Pack_Voltage] -> Rinehart Inverter Thermal Model/1(In1)
  [Inverter_Cool_in] -> Rinehart Inverter Thermal Model/3(In3)
  [Motor_Cool_in] -> EMRAX Motor Thermal Model/4(Temp_cool_RAD_out [K])
  "Limit Torque/Power if neccessary for thermal "/1(Out1) -> Out1/1  "Limited_Motor_Torque"
  "Limit Torque/Power if neccessary for thermal "/2(Out2) -> Out2/1  "P_requested_from_Pack"

== system BuckeyeCurrent_Simulation/Motorcycle Model/Transmission/Gearbox  ==
  note: This will become true as motor nears it top speed and torque drops
  In1 : Inport
  EM Max Torque Curve : Lookup  InputValues=EM.N_RPM  Table=EM.T_max_Peak  LookUpMeth=Interpolation-Use End Values  SaturateOnIntegerOverflow=on
  EM Max Torque Curve1 : Lookup  InputValues=EM.N_RPM  Table=EM.T_max_Peak  LookUpMeth=Interpolation-Use End Values  SaturateOnIntegerOverflow=on
  Multiply : Product  Inputs=***
  Product : Product
  Product1 : Product
  Sum : Sum  Inputs=+-
  Switch : Switch  Criteria=u2 > Threshold
  Out2 : Outport
  Out1 : Outport  Port=2
  tag scope: Final_Drive_Ratio=global
  wires:
  [Final_Drive_Eff] -> Multiply/3
  Multiply/1 -> Out1/1  "Wheel Torque"
  In1/1 -> Multiply/2  "Motor Torque"
  [Final_Drive_Ratio_1st] -> Switch/3  "Final Drive Ratio"
  [Final_Drive_Ratio_2nd] -> Switch/1
  Sum/1 -> Switch/2  "When T_second > T_First (at wheel), Switch gears"
  Switch/1 -> [Final_Drive_Ratio], Out2/1, Multiply/1  "Final Drive Ratio"
  [EM_RPM_2nd] -> EM Max Torque Curve1/1
  [EM_RPM_1st] -> EM Max Torque Curve/1
  EM Max Torque Curve1/1 -> Product/2
  [Final_Drive_Ratio_2nd] -> Product/1
  EM Max Torque Curve/1 -> Product1/1
  [Final_Drive_Ratio_1st] -> Product1/2
  Product1/1 -> Sum/2
  Product/1 -> Sum/1

== system BuckeyeCurrent_Simulation/Road Loads/Vehicle Loads/Aerodynamic  Drag ==
  Constant : Constant  Value=0.5
  Drag force =1/2*row_a*Cd*Af*v2 : Product  Inputs=4  RndMeth=Zero
  Sum : Sum  Inputs=|++
  drag_v1 : Math  Operator=pow  SaturateOnIntegerOverflow=on
  square : Constant  Value=2
  Drag Power : Outport
  wires:
  square/1 -> drag_v1/2
  Constant/1 -> Drag force =1/2*row_a*Cd*Af*v2/1
  [Cda] -> Drag force =1/2*row_a*Cd*Af*v2/3
  [Row_Air] -> Drag force =1/2*row_a*Cd*Af*v2/2
  Drag force =1/2*row_a*Cd*Af*v2/1 -> Drag Power/1  "Drag_Force (N)"
  [Vehicle_Velocity_ms] -> Sum/1
  Sum/1 -> drag_v1/1
  [Wind_Speed] -> Sum/2
  drag_v1/1 -> Drag force =1/2*row_a*Cd*Af*v2/4

== system BuckeyeCurrent_Simulation/Road Loads/Vehicle Loads/Grade Force ==
  note: If grade force is NaN, apply 0 force, otherwise export grade force
  Constant : Constant  Value=0
  Divide : Product  Inputs=*/
  Elevation : Lookup  InputValues=Elevation_Profile.distance  Table=Elevation_Profile.elevation  LookUpMeth=Interpolation-Use End Values  SaturateOnIntegerOverflow=on
  Fcn : Fcn  Expr=sin(u)
  Fcn1 : Fcn  Expr=atan(u(1))
  Grade Force = M*g*sin(road_grade) : Product  Inputs=3  RndMeth=Zero
  Memory : Memory
  Past Elevation : Lookup  InputValues=Elevation_Profile.distance  Table=Elevation_Profile.elevation  LookUpMeth=Interpolation-Use End Values  SaturateOnIntegerOverflow=on
  Relational Operator : RelationalOperator  Operator=isNaN  OutDataTypeStr=boolean  RndMeth=Simplest
  Sum : Sum  Inputs=+-
  Sum1 : Sum  Inputs=-+
  Switch : Switch  Threshold=1
  gravity : Constant  Value=9.81
  Drag Power : Outport
  wires:
  Fcn1/1 -> Fcn/1
  [Mass] -> Grade Force = M*g*sin(road_grade)/1
  gravity/1 -> Grade Force = M*g*sin(road_grade)/2
  Divide/1 -> Fcn1/1
  Past Elevation/1 -> Sum/2
  Memory/1 -> Sum1/1, Past Elevation/1
  Sum/1 -> Divide/1  "Elevation change"
  Elevation/1 -> Sum/1
  [Distance_Total_m] -> Sum1/2, Memory/1, Elevation/1
  Sum1/1 -> Divide/2  "Distance Change"
  Fcn/1 -> Grade Force = M*g*sin(road_grade)/3
  Switch/1 -> Drag Power/1  "Grade_Force (N)"
  Grade Force = M*g*sin(road_grade)/1 -> Switch/3, Relational Operator/1  "Grade_Force(N)"
  Relational Operator/1 -> Switch/2
  Constant/1 -> Switch/1

== system BuckeyeCurrent_Simulation/Road Loads/Vehicle Loads/Roll Force ==
  note: Create a more accurate estimate later (Cossalter has formulas)
  Aprrox. Rolling Resistance Force : Constant  Value=0.02
  Gravity (m/s2) : Constant  Value=9.81
  Product : Product  Inputs=3
  Power_roll : Outport
  wires:
  Product/1 -> Power_roll/1  "Roll_Force (N)"
  [Mass] -> Product/1
  Gravity (m/s2)/1 -> Product/2
  Aprrox. Rolling Resistance Force/1 -> Product/3

== system BuckeyeCurrent_Simulation/Motorcycle Model/Battery Pack/Current Lim, 1st Order ECM, Thermal, Regen/Battery Parameters Calculation ==
  note: if I<0 --> CHARGE
  note: if I>0 --> DISCHARGE
  current1 : Inport
  Demux : Demux  Outputs=3
  OCV Calculation for Battery : Subsystem
      mask Display:
      | color('blue');
      | fprintf('OCV Calculation')
  "R0, C1, R1 Calculation for Battery" : Subsystem
      mask Display:
      | color('blue');
      | fprintf('R0, C1, R1, Calculation', 17)
  SOC Calculation for Battery : Subsystem
      mask Display:
      | color('blue');
      | fprintf('SOC Calculation')
  Switch CHARGE OR DISCHARGE : Switch  Criteria=u2 > Threshold
  tag scope: C1=global, R0=global, R1=global
  wires:
  Demux/3 -> [C1]
  Demux/2 -> [R1]
  Demux/1 -> [R0]
  Switch CHARGE OR DISCHARGE/1 -> Demux/1
  [BAT_Ch] -> Switch CHARGE OR DISCHARGE/3
  [BAT_DisCh] -> Switch CHARGE OR DISCHARGE/1
  current1/1 -> Switch CHARGE OR DISCHARGE/2, SOC Calculation for Battery/1(In1)

== system BuckeyeCurrent_Simulation/Motorcycle Model/Battery Pack/Current Lim, 1st Order ECM, Thermal, Regen/Battery to Cell ==
  In1 : Inport
  Divide : Product  Inputs=*/
  Out1 : Outport
  tag scope: I_Cell_Request=global
  wires:
  In1/1 -> Divide/1  "I_Bat_Req"
  [cellParallelCount] -> Divide/2
  Divide/1 -> [I_Cell_Request], Out1/1  "I_Cell_Req"

== system BuckeyeCurrent_Simulation/Motorcycle Model/Battery Pack/Current Lim, 1st Order ECM, Thermal, Regen/Cell ==
  In2 : Inport
  " " : Sum  Inputs=+-
  Add : Sum  Inputs=+--
  I*R0 : Product  RndMeth=Zero
  I/C1 : Product  Inputs=*/
  "VC_dot * C1 " : Product  RndMeth=Zero
  V_c : Integrator
  Vc/R1*C1 : Product  Inputs=//*
  dvc/dt : Sum  Inputs=+-
  Out1 : Outport
  Out2 : Outport  Port=2
  tag scope: I_R1=global
  wires:
  I*R0/1 -> Add/2
  [R0] -> I*R0/1  "R0"
  [OCV] -> Add/1  "OCV"
  In2/1 -> I/C1/1, " "/1, Out2/1, I*R0/2
  Add/1 -> Out1/1  "V_Cell"
  dvc/dt/1 -> "VC_dot * C1 "/2, V_c/1
  I/C1/1 -> dvc/dt/1
  [C1] -> I/C1/2, Vc/R1*C1/2, "VC_dot * C1 "/1  "C1"
  V_c/1 -> Vc/R1*C1/3, Add/3  "Vc"
  Vc/R1*C1/1 -> dvc/dt/2
  [R1] -> Vc/R1*C1/1  "R1"
  "VC_dot * C1 "/1 -> " "/2
  " "/1 -> [I_R1]  "I_R1"

== system BuckeyeCurrent_Simulation/Motorcycle Model/Battery Pack/Current Lim, 1st Order ECM, Thermal, Regen/Cell to Batt ==
  In1 : Inport
  In2 : Inport  Port=2
  multiply1 : Product  Inputs=**
  multiply2 : Product  Inputs=**
  multiply3 : Product  Inputs=**
  Out1 : Outport
  Out3 : Outport  Port=2
  tag scope: I_Batt=global, V_Batt=global
  wires:
  [cellSeriesCount] -> multiply1/1
  multiply1/1 -> [V_Batt], Out1/1, multiply3/1  "V_Batt"
  In1/1 -> multiply1/2
  In2/1 -> multiply2/1
  [cellParallelCount] -> multiply2/2
  multiply2/1 -> multiply3/2, [I_Batt]  "I_Batt"
  multiply3/1 -> Out3/1  "P_Batt"

== system BuckeyeCurrent_Simulation/Motorcycle Model/Battery Pack/Current Lim, 1st Order ECM, Thermal, Regen/Thermal Dynamics ==
  " 1" : Sum  Inputs=+-
  " 2" : Sum  Inputs=-+
  A : Constant  Value=BATT_THERMAL.A
  Divide : Product  Inputs=**/
  Integrator : Integrator  InitialConditionSource=external  InitialCondition=ambTemp_K
  Pack Heat Generation : Subsystem
  Product : Product  Inputs=4  RndMeth=Zero
  h : Constant  Value=BATT_THERMAL.h
  m*c : Product  RndMeth=Zero
  tag scope: T_Batt=global
  wires:
  Pack Heat Generation/1(Out1) -> " 1"/1
  [ambTemp_K] -> " 2"/1
  Integrator/1 -> [T_Batt], " 2"/2  "T_Batt"
  Product/1 -> " 1"/2
  A/1 -> Product/3
  h/1 -> Product/2
  " 2"/1 -> Product/4
  " 1"/1 -> Divide/2
  Divide/1 -> Integrator/1
  [ambTemp_K] -> Integrator/2
  [totalCellCount] -> Product/1, Divide/1
  [BatteryPack_mass_g] -> m*c/1
  [BatteryPack_c] -> m*c/2
  m*c/1 -> Divide/3

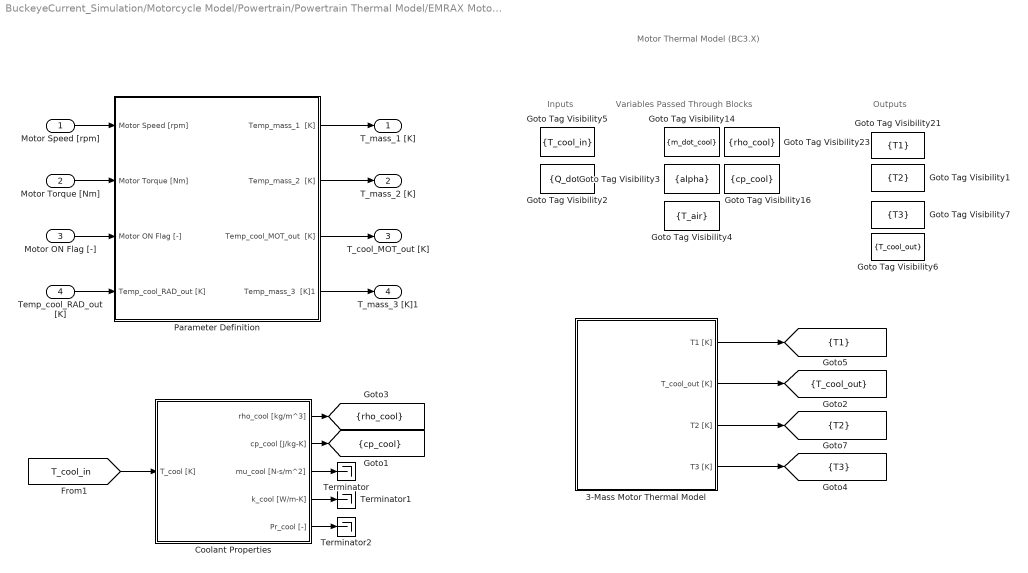
== system BuckeyeCurrent_Simulation/Motorcycle Model/Powertrain/Powertrain Thermal Model/EMRAX Motor Thermal Model ==
  note: Variables Passed Through Blocks
  note: Inputs
  note: Motor Thermal Model
      | (BC3.X)
  note: Outputs
  Motor Speed [rpm] : Inport
  Motor Torque [Nm] : Inport  Port=2
  Motor ON Flag [-] : Inport  Port=3
  Temp_cool_RAD_out [K] : Inport  Port=4
  3-Mass Motor Thermal Model : Subsystem
  Coolant Properties : Subsystem
  Goto Tag Visibility1 : GotoTagVisibility  GotoTag=T2
  Goto Tag Visibility14 : GotoTagVisibility  GotoTag=m_dot_cool
  Goto Tag Visibility16 : GotoTagVisibility  GotoTag=cp_cool
  Goto Tag Visibility2 : GotoTagVisibility  GotoTag=Q_dot
  Goto Tag Visibility21 : GotoTagVisibility  GotoTag=T1
  Goto Tag Visibility23 : GotoTagVisibility  GotoTag=rho_cool
  Goto Tag Visibility3 : GotoTagVisibility  GotoTag=alpha
  Goto Tag Visibility4 : GotoTagVisibility  GotoTag=T_air
  Goto Tag Visibility5 : GotoTagVisibility  GotoTag=T_cool_in
  Goto Tag Visibility6 : GotoTagVisibility  GotoTag=T_cool_out
  Goto Tag Visibility7 : GotoTagVisibility  GotoTag=T3
  Parameter Definition : Subsystem
  Terminator : Terminator
  Terminator1 : Terminator
  Terminator2 : Terminator
  T_mass_1 [K] : Outport
  T_mass_2 [K] : Outport  Port=2
  T_cool_MOT_out [K] : Outport  Port=3
  T_mass_3 [K]1 : Outport  Port=4
  tag scope: T1=scoped, T2=scoped, T3=scoped, T_cool_out=scoped, cp_cool=scoped, rho_cool=scoped
  wires:
  Coolant Properties/1(rho_cool [kg/m^3]) -> [rho_cool]
  Coolant Properties/2(cp_cool [J/kg-K]) -> [cp_cool]
  [T_cool_in] -> Coolant Properties/1(T_cool [K])
  Coolant Properties/3(mu_cool [N-s/m^2]) -> Terminator/1
  Coolant Properties/4(k_cool [W/m-K]) -> Terminator1/1
  Coolant Properties/5(Pr_cool [-]) -> Terminator2/1
  3-Mass Motor Thermal Model/1(T1 [K]) -> [T1]
  3-Mass Motor Thermal Model/3(T2 [K]) -> [T2]
  Motor Torque [Nm]/1 -> Parameter Definition/2(Motor Torque [Nm])
  Motor ON Flag [-]/1 -> Parameter Definition/3(Motor ON Flag [-])
  Temp_cool_RAD_out [K]/1 -> Parameter Definition/4(Temp_cool_RAD_out [K])
  Parameter Definition/2(Temp_mass_2  [K]) -> T_mass_2 [K]/1
  Motor Speed [rpm]/1 -> Parameter Definition/1(Motor Speed [rpm])
  3-Mass Motor Thermal Model/2(T_cool_out [K]) -> [T_cool_out]
  Parameter Definition/3(Temp_cool_MOT_out  [K]) -> T_cool_MOT_out [K]/1
  Parameter Definition/1(Temp_mass_1  [K]) -> T_mass_1 [K]/1
  Parameter Definition/4(Temp_mass_3  [K]1) -> T_mass_3 [K]1/1
  3-Mass Motor Thermal Model/4(T3 [K]) -> [T3]

== system BuckeyeCurrent_Simulation/Motorcycle Model/Powertrain/Powertrain Thermal Model/Limit Torque//Power if neccessary for thermal  ==
  Out1 : Outport
  Out2 : Outport  Port=2
  wires:
  ? -> Out1/1  "Motor Torque"
  ? -> Out2/1  "Inverter_P_Request"

== system BuckeyeCurrent_Simulation/Motorcycle Model/Powertrain/Powertrain Thermal Model/Radiator Thermal Model ==
  T_cool_in [K] : Inport
  q_cool_in [m^3/s] : Inport  Port=2
  T_air [K] : Inport  Port=3
  V_face [m/s] : Inport  Port=4
  Air Properties : Subsystem
  Coolant Properties : Subsystem
  Goto Tag Visibility10 : GotoTagVisibility  GotoTag=rho_air
  Goto Tag Visibility3 : GotoTagVisibility  GotoTag=rho_cool
  Goto Tag Visibility4 : GotoTagVisibility  GotoTag=cp_cool
  Goto Tag Visibility7 : GotoTagVisibility  GotoTag=mu_cool
  Goto Tag Visibility8 : GotoTagVisibility  GotoTag=k_cool
  Goto Tag Visibility9 : GotoTagVisibility  GotoTag=Pr_cool
  Reduced Radiator Thermal Model (1 Node - 1 Mass) : Subsystem
  Terminator : Terminator
  T_cool_out [K] : Outport
  Q_dot_RAD [W] : Outport  Port=2
  tag scope: Pr_cool=scoped, cp_cool=scoped, k_cool=scoped, mu_cool=scoped, rho_air=scoped, rho_cool=scoped
  wires:
  Coolant Properties/4(k_cool [W/m-K]) -> [k_cool]
  Air Properties/1(rho_air [kg/m^3]) -> [rho_air]
  Reduced Radiator Thermal Model (1 Node - 1 Mass)/2(Q_dot_RAD [W]) -> Q_dot_RAD [W]/1
  Coolant Properties/2(cp_cool [J/kg-K]) -> [cp_cool]
  T_air [K]/1 -> Reduced Radiator Thermal Model (1 Node - 1 Mass)/3(T_air [K]), Air Properties/1(T_air_in [K])
  Reduced Radiator Thermal Model (1 Node - 1 Mass)/1(T_cool_out [K]) -> T_cool_out [K]/1
  T_cool_in [K]/1 -> Reduced Radiator Thermal Model (1 Node - 1 Mass)/1(T_cool_in [K]), Coolant Properties/1(T_cool [K])
  Air Properties/2(cp_air [J/kg-K]) -> Terminator/1
  q_cool_in [m^3/s]/1 -> Reduced Radiator Thermal Model (1 Node - 1 Mass)/2(q_cool_in [m^3/s])
  V_face [m/s]/1 -> Reduced Radiator Thermal Model (1 Node - 1 Mass)/4(V_face [m/s])
  Coolant Properties/5(Pr_cool [-]) -> [Pr_cool]
  Coolant Properties/1(rho_cool [kg/m^3]) -> [rho_cool]
  Coolant Properties/3(mu_cool [N-s/m^2]) -> [mu_cool]

== system BuckeyeCurrent_Simulation/Motorcycle Model/Powertrain/Powertrain Thermal Model/Rinehart Inverter Thermal Model ==
  In1 : Inport
  In2 : Inport  Port=2
  In3 : Inport  Port=3
  Coolant Properties : Subsystem
  Inverter Thermal Model : Subsystem
  Terminator : Terminator
  Terminator1 : Terminator
  Terminator2 : Terminator
  Out1 : Outport
  Out2 : Outport  Port=2
  Out3 : Outport  Port=3
  tag scope: cp_cool=scoped, rho_cool=scoped
  wires:
  Coolant Properties/3(mu_cool [N-s/m^2]) -> Terminator/1
  Coolant Properties/5(Pr_cool [-]) -> Terminator2/1
  Coolant Properties/1(rho_cool [kg/m^3]) -> [rho_cool]
  Coolant Properties/4(k_cool [W/m-K]) -> Terminator1/1
  Coolant Properties/2(cp_cool [J/kg-K]) -> [cp_cool]
  Inverter Thermal Model/2(Out2) -> Out2/1  "Module Case Temp"
  In1/1 -> Inverter Thermal Model/1(In1)  "Pack Voltage"
  Inverter Thermal Model/3(Out3) -> Out3/1  "Coolant out Temp"
  Inverter Thermal Model/1(Out1) -> Out1/1  "Electrical Device Temps"
  In3/1 -> Coolant Properties/1(T_cool [K]), Inverter Thermal Model/3(In3)  "Coolant Temp, in"
  In2/1 -> Inverter Thermal Model/2(In2)  "RMS_Current"

== system BuckeyeCurrent_Simulation/Motorcycle Model/Battery Pack/Current Lim, 1st Order ECM, Thermal, Regen/Battery Parameters Calculation/OCV Calculation for Battery ==
  SoC vs. OCV : Lookup  InputValues=BATT_OCV.SoC  Table=BATT_OCV.OCV  LookUpMeth=Interpolation-Use End Values
  tag scope: OCV=global
  wires:
  [SOC_Batt] -> SoC vs. OCV/1
  SoC vs. OCV/1 -> [OCV]

== system BuckeyeCurrent_Simulation/Motorcycle Model/Battery Pack/Current Lim, 1st Order ECM, Thermal, Regen/Battery Parameters Calculation/R0, C1, R1 Calculation for Battery ==
  C1 Ch : Lookup2D  RowIndex=BATT_ELEC.temp_part  ColumnIndex=BATT_ELEC.soc_part  Table=BATT_ELEC.C1c  LookUpMeth=Interpolation-Use End Values
  C1 Disch : Lookup2D  RowIndex=BATT_ELEC.temp_part  ColumnIndex=BATT_ELEC.soc_part  Table=BATT_ELEC.C1d  LookUpMeth=Interpolation-Use End Values
  Constant : Constant  Value=273
  Math Reciprocal : Math  Operator=reciprocal  SaturateOnIntegerOverflow=on
  Mux : Mux  Inputs=3
  Mux1 : Mux  Inputs=3
  Product : Product
  Product1 : Product
  R0 Disch : Lookup2D  RowIndex=BATT_ELEC.temp_part  ColumnIndex=BATT_ELEC.soc_part  Table=BATT_ELEC.R0d  LookUpMeth=Interpolation-Use End Values
  R0 ch : Lookup2D  RowIndex=BATT_ELEC.temp_part  ColumnIndex=BATT_ELEC.soc_part  Table=BATT_ELEC.R0c  LookUpMeth=Interpolation-Use End Values
  R1 Ch : Lookup2D  RowIndex=BATT_ELEC.temp_part  ColumnIndex=BATT_ELEC.soc_part  Table=BATT_ELEC.R1c  LookUpMeth=Interpolation-Use End Values
  R1 Disch : Lookup2D  RowIndex=BATT_ELEC.temp_part  ColumnIndex=BATT_ELEC.soc_part  Table=BATT_ELEC.R1d  LookUpMeth=Interpolation-Use End Values
  Sum : Sum  Inputs=-+|
  tag scope: BAT_Ch=global, BAT_DisCh=global
  wires:
  Sum/1 -> C1 Ch/1, R1 Ch/1, R0 ch/1, C1 Disch/1, R1 Disch/1, R0 Disch/1
  [SOC_Batt] -> C1 Ch/2, R1 Ch/2, R0 ch/2, C1 Disch/2, R1 Disch/2, R0 Disch/2
  Mux1/1 -> Product1/2
  Constant/1 -> Sum/1
  [T_Batt] -> Sum/2
  R0 Disch/1 -> Mux/1
  C1 Disch/1 -> Mux/3
  R1 Disch/1 -> Mux/2
  R0 ch/1 -> Mux1/1
  R1 Ch/1 -> Mux1/2
  C1 Ch/1 -> Mux1/3
  Product/1 -> [BAT_DisCh]
  Mux/1 -> Product/1
  [cellParallelCount] -> Math Reciprocal/1
  Math Reciprocal/1 -> Product/2, Product1/1
  Product1/1 -> [BAT_Ch]

== system BuckeyeCurrent_Simulation/Motorcycle Model/Battery Pack/Current Lim, 1st Order ECM, Thermal, Regen/Battery Parameters Calculation/SOC Calculation for Battery ==
  In1 : Inport
  Integrator : Integrator  InitialConditionSource=external  InitialCondition=soc0  LimitOutput=on  UpperSaturationLimit=100  LowerSaturationLimit=0
  Math Reciprocal : Math  Operator=reciprocal  SaturateOnIntegerOverflow=on
  Product1 : Product  Inputs=3  RndMeth=Zero
  Product2 : Product  RndMeth=Zero
  SoC % : Gain  Gain=100
  capacity : Constant  Value=-1/(3600)
  tag scope: SOC_Batt=global
  wires:
  Product1/1 -> SoC %/1
  capacity/1 -> Product1/1
  Math Reciprocal/1 -> Product1/3
  In1/1 -> Product1/2
  Integrator/1 -> [SOC_Batt]  "SoC_Batt"
  SoC %/1 -> Integrator/1
  [soc0] -> Integrator/2
  [cellCapacity] -> Product2/1
  [cellParallelCount] -> Product2/2
  Product2/1 -> Math Reciprocal/1

== system BuckeyeCurrent_Simulation/Motorcycle Model/Battery Pack/Current Lim, 1st Order ECM, Thermal, Regen/Thermal Dynamics/Pack Heat Generation ==
  Add : Sum
  I1_cell^2 x R1 : Product  RndMeth=Zero
  I_cell^2 x R0 : Product  RndMeth=Zero
  I_cell^2 x R1 : Product  Inputs=3  RndMeth=Zero
  Math Function : Math  Operator=square  SaturateOnIntegerOverflow=on
  Math Function1 : Math  Operator=square  SaturateOnIntegerOverflow=on
  Memory{,1..3} (4 alike) : Memory
  Out1 : Outport
  tag scope: P_Heat_Batt=global
  wires:
  [R0] -> Memory1/1
  [I_Cell_Request] -> Memory/1
  Math Function/1 -> I_cell^2 x R0/1
  [I_R1] -> Memory2/1
  [R1] -> Memory3/1
  I1_cell^2 x R1/1 -> Add/2
  I_cell^2 x R0/1 -> Add/1
  Add/1 -> I_cell^2 x R1/1  "Q_dot_Cell"
  I_cell^2 x R1/1 -> [P_Heat_Batt], Out1/1  "Q_dot_Batt"
  [cellParallelCount] -> I_cell^2 x R1/2
  [cellSeriesCount] -> I_cell^2 x R1/3
  Math Function1/1 -> I1_cell^2 x R1/1
  Memory/1 -> Math Function/1
  Memory1/1 -> I_cell^2 x R0/2
  Memory2/1 -> Math Function1/1
  Memory3/1 -> I1_cell^2 x R1/2

== system BuckeyeCurrent_Simulation/Motorcycle Model/Powertrain/Powertrain Thermal Model/EMRAX Motor Thermal Model/3-Mass Motor Thermal Model ==
  "Mass 1 : Stator Block" : Subsystem
  Mass 2 :Rotor Block : Subsystem
  "Mass 3 : Motor Mounting" : Subsystem
  T1 [K] : Outport
  T_cool_out [K] : Outport  Port=2
  T2 [K] : Outport  Port=3
  T3 [K] : Outport  Port=4
  wires:
  [Q_dot] -> Mass 2 :Rotor Block/1(Q_dot_heat [W]), "Mass 1 : Stator Block"/1(Q_dot_heat [W])
  Mass 2 :Rotor Block/1(T2 [K]) -> "Mass 3 : Motor Mounting"/1("T2 "), "Mass 1 : Stator Block"/2(T2 [K]), T2 [K]/1
  [T_cool_in] -> "Mass 1 : Stator Block"/3(T_cool_in [K])
  "Mass 1 : Stator Block"/1(T1 [K]) -> Mass 2 :Rotor Block/2(T1), T1 [K]/1
  [m_dot_cool] -> "Mass 1 : Stator Block"/4(m_dot_cool [kg/s])
  "Mass 1 : Stator Block"/2(T_cool_out) -> T_cool_out [K]/1
  "Mass 3 : Motor Mounting"/1(T3 [K]) -> Mass 2 :Rotor Block/3(T3), T3 [K]/1
